simulink model "Bicycle_model_nonlinear_constrained"  (R2020b)
settings: Solver=ode15s  StartTime=0.0  StopTime=10.0  RelTol=1e-3
InitFcn:
  | mdl = 'Bicycle_model_nonlinear_constrained';
  | 
  | wks = get_param(mdl, 'ModelWorkspace');
  | 
  | vals_struct_front = load('lateral_data_lut_FRONT.mat');
  | sa_x_front = vals_struct_front.sa_x;
  | load_y_front = vals_struct_front.load_y;
  | %sa_x_front = sa_x_front'*ones(1, length(load_y_front));
  | load_y_front = flip(load_y_front);
  | %load_y_front = ones(size(sa_x_front, 1), 1)*load_y_front;
  | lateral_coeff_front = vals_struct_front.lat_coeff;
  | lateral_coeff_front = fliplr(lateral_coeff_front);
  | aligning_torque_front = vals_struct_front.aligning_torque;
  | aligning_torque_front = fliplr(aligning_torque_front);
  | assignin(wks, 'sa_x_front', sa_x_front);
  | assignin(wks, 'load_y_front', load_y_front);
  | assignin(wks, 'lateral_coeff_front', lateral_coeff_front);
  | assignin(wks, 'aligning_torque_front', aligning_torque_front);
  | 
  | vals_struct_rear = load('lateral_data_lut_REAR.mat');
  | sa_x_rear = vals_struct_rear.sa_x;
  | load_y_rear = vals_struct_rear.load_y;
  | %sa_x_rear = sa_x_rear'*ones(1, length(load_y_rear));
  | load_y_rear = flip(load_y_rear);
  | %load_y_rear = ones(size(sa_x_rear, 1), 1)*load_y_rear;
  | lateral_coeff_rear = vals_struct_rear.lat_coeff;
  | lateral_coeff_rear = fliplr(lateral_coeff_rear);
  | aligning_torque_rear = vals_struct_rear.aligning_torque;
  | aligning_torque_rear = fliplr(aligning_torque_rear);
  | assignin(wks, 'sa_x_rear', sa_x_rear);
  | assignin(wks, 'load_y_rear', load_y_rear);
  | assignin(wks, 'lateral_coeff_rear', lateral_coeff_rear);
  | assignin(wks, 'aligning_torque_rear', aligning_torque_rear);
model workspace (MAT data in the model file):
  Gravity = Simulink.Parameter
  Gravity.Value = 9.81
  Gravity.DataType = 'auto'
  Gravity.DocUnits = 'N/kg'
  Gravity.Dimensions = [1 1]
  Mass = Simulink.Parameter
  Mass.Value = 285
  Mass.DataType = 'auto'
  Mass.Dimensions = [1 1]
  Weight_dist = Simulink.Parameter
  Weight_dist.Value = 0.6
  Weight_dist.DataType = 'auto'
  Weight_dist.Dimensions = [1 1]
  Wheelbase = Simulink.Parameter
  Wheelbase.Value = 1.53
  Wheelbase.DataType = 'auto'
  Wheelbase.Dimensions = [1 1]
  aligning_torque_front = [-41.5540960755 -41.5662624888 -41.5807188002 -41.5975229416 -41.6167266751 -41.6383748526 -41.6625046744 -41.6891449542 -41.7183154014 -41.7500259272 -41.7842759867 -41.8210539664 ... (18361 elements, 301x61)]
  aligning_torque_rear = [-18.1434786147 -17.5139711055 -16.8077956028 -16.0208528857 -15.1497738315 -14.1923038543 -13.1478032051 -12.0178890979 -10.8072479379 -9.52464615821 -8.18416446104 -6.80666977097 ... (18361 elements, 301x61)]
  lateral_coeff_front = [-2.08355014577 -2.08846565202 -2.09327995784 -2.09799213228 -2.10260121652 -2.10710622309 -2.11150613503 -2.11579990501 -2.11998645448 -2.1240646727 -2.12803341584 -2.13189150601 ... (18361 elements, 301x61)]
  lateral_coeff_rear = [-2.53828292724 -2.53442829982 -2.53054773666 -2.5266407201 -2.52270671872 -2.51874518685 -2.51475556411 -2.51073727486 -2.50668972773 -2.50261231503 -2.49850441218 -2.49436537715 ... (18361 elements, 301x61)]
  load_y_front = [-1200 -1180 -1160 -1140 -1120 -1100 -1080 -1060 -1040 -1020 -1000 -980 -960 -940 -920 -900 -880 -860 -840 -820 -800 -780 -760 -740 -720 -700 -680 -660 -640 -620 -600 -580 -560 -540 -520 -500 -480 -460 -440 -420 -400 -380 -360 -340 -320 -300 -280 -260 -240 -220 -200 -180 -160 -140 -120 -100 -80 -60 -40 -20 0]
  load_y_rear = [-1200 -1180 -1160 -1140 -1120 -1100 -1080 -1060 -1040 -1020 -1000 -980 -960 -940 -920 -900 -880 -860 -840 -820 -800 -780 -760 -740 -720 -700 -680 -660 -640 -620 -600 -580 -560 -540 -520 -500 -480 -460 -440 -420 -400 -380 -360 -340 -320 -300 -280 -260 -240 -220 -200 -180 -160 -140 -120 -100 -80 -60 -40 -20 0]
  sa_x_front = [-0.261799387799 -0.260054058547 -0.258308729295 -0.256563400043 -0.254818070791 -0.253072741539 -0.251327412287 -0.249582083035 -0.247836753783 -0.246091424531 -0.244346095279 -0.242600766027 ... (301 elements, 1x301)]
  sa_x_rear = [-0.261799387799 -0.260054058547 -0.258308729295 -0.256563400043 -0.254818070791 -0.253072741539 -0.251327412287 -0.249582083035 -0.247836753783 -0.246091424531 -0.244346095279 -0.242600766027 ... (301 elements, 1x301)]
libraries: simulink_extras x4
(part 1 of 2)
settings Model: OrderedModelArguments=off  Creator=yafta  LastModifiedBy=Matthew

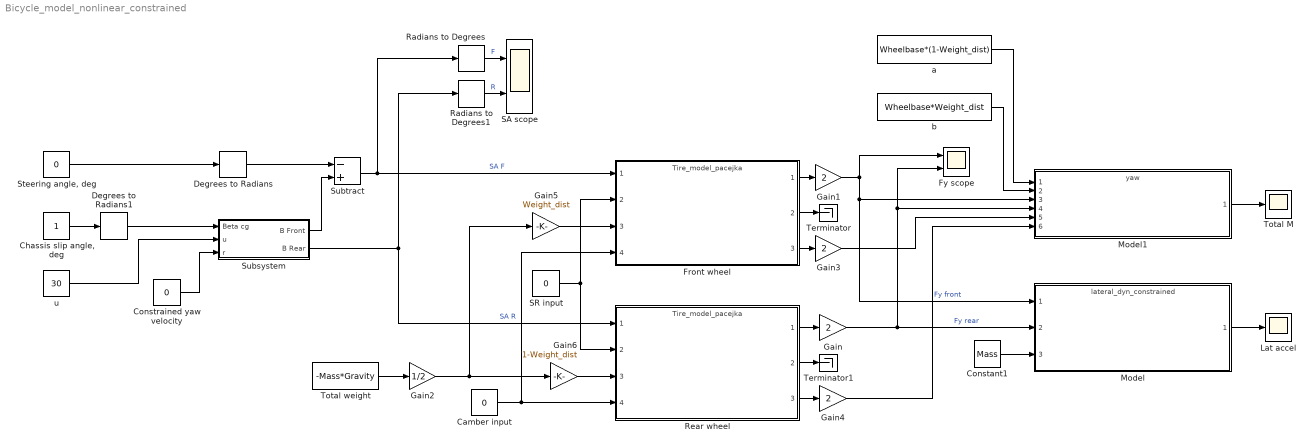
== system Bicycle_model_nonlinear_constrained ==
  Camber input : Constant  Value=0
  "Chassis slip angle, deg" : Constant
  Constant1 : Constant  Value=Mass
  Constrained yaw velocity : Constant  Value=0
  Degrees to Radians : simulink_extras/Transformations/Degrees to Radians
  Degrees to Radians1 : simulink_extras/Transformations/Degrees to Radians
  Front wheel : ModelReference  ModelNameDialog=Tire_model_pacejka.slx  UsingDefaultArgumentValue=0,0  SimulationMode=Normal  ModelReferenceVersion=2.9
  Fy scope : Scope  NumInputPorts=2
  Gain{,1,3..4} (4 alike) : Gain  Gain=2
  Gain2 : Gain  Gain=1/2
  Gain5 : Gain  Gain=Weight_dist
  Gain6 : Gain  Gain=1-Weight_dist
  Lat accel : Scope
  Model : ModelReference  ModelNameDialog=lateral_dyn_constrained.slx  SimulationMode=Normal  ModelReferenceVersion=2.3
  Model1 : ModelReference  ModelNameDialog=yaw.slx  SimulationMode=Normal  ModelReferenceVersion=2.11
  Radians to Degrees : simulink_extras/Transformations/Radians to Degrees
  Radians to Degrees1 : simulink_extras/Transformations/Radians to Degrees
  Rear wheel : ModelReference  ModelNameDialog=Tire_model_pacejka.slx  UsingDefaultArgumentValue=0,0  SimulationMode=Normal  ModelReferenceVersion=2.9
  SA scope : Scope  NumInputPorts=2
  SR input : Constant  Value=0
  "Steering angle, deg" : Constant  Value=0
  Subsystem : Subsystem
  Subtract : Sum  Inputs=-+
  Terminator : Terminator
  Terminator1 : Terminator
  Total M : Scope
  Total weight : Constant  Value=-Mass*Gravity
  a : Constant  Value=Wheelbase*(1-Weight_dist)
  b : Constant  Value=Wheelbase*Weight_dist
  u : Constant  Value=30
  wires:
  Rear wheel/2 -> Terminator1/1
  Gain6/1 -> Rear wheel/3
  Subtract/1 -> Front wheel/1, Radians to Degrees/1  "SA F"
  Constant1/1 -> Model/3
  Front wheel/2 -> Terminator/1
  Degrees to Radians/1 -> Subtract/1
  a/1 -> Model1/1
  Constrained yaw velocity/1 -> Subsystem/3(r)
  Gain2/1 -> Gain6/1, Gain5/1
  Gain5/1 -> Front wheel/3
  Camber input/1 -> Rear wheel/4, Front wheel/4
  Gain3/1 -> Model1/5
  u/1 -> Subsystem/2(u)
  Model1/1 -> Total M/1
  Rear wheel/1 -> Gain/1
  SR input/1 -> Front wheel/2, Rear wheel/2
  Radians to Degrees1/1 -> SA scope/2  "R"
  Front wheel/1 -> Gain1/1
  Degrees to Radians1/1 -> Subsystem/1(Beta cg)
  Front wheel/3 -> Gain3/1
  Gain4/1 -> Model1/6
  Subsystem/2(B Rear) -> Radians to Degrees1/1, Rear wheel/1  "SA R"
  b/1 -> Model1/2
  Total weight/1 -> Gain2/1
  Subsystem/1(B Front) -> Subtract/2
  Model/1 -> Lat accel/1
  Rear wheel/3 -> Gain4/1
  Gain/1 -> Fy scope/2, Model1/4, Model/2  "Fy rear"
  "Chassis slip angle, deg"/1 -> Degrees to Radians1/1
  Radians to Degrees/1 -> SA scope/1  "F"
  "Steering angle, deg"/1 -> Degrees to Radians/1
  Gain1/1 -> Model/1, Model1/3, Fy scope/1  "Fy front"
